simulink model "coupled_model"  (R2025b)
settings: Solver=ode4  StartTime=0.0  StopTime=20  FixedStep=0.01  RelTol=1e-3
InitFcn:
  | setup;
values from neighbouring files (symbols this model uses):
  K_GAIN = 1.0    (= 1)    [setup.m]
  N = 1000    [plot_out.m]    (also in setup.m)
  P_GAIN = 200.0    (= 200)    [setup.m]
  phase_offsets = [PHASE_OFFSET_RAD, -PHASE_OFFSET_RAD]    [setup.m]
  robot_params = struct()    [setup.m]
undefined symbols (not defined in the file or in its folder): tables1, tables2, X, Y, Z
libraries: sm_lib x30, nesl_utility x16
settings Model: Creator=mahdi  LastModifiedBy=root
settings SolverCC: AlgebraicLoopSolver=TrustRegion
settings DebuggingCC: UnconnectedInputMsg=warning  UnconnectedOutputMsg=warning  UnconnectedLineMsg=warning
settings ModelReferenceCC: EnableRefExpFcnMdlSchedulingChecks=on
settings RTWCC: GPUComputeCapability=3.5  DLArmComputeVersion=19.05

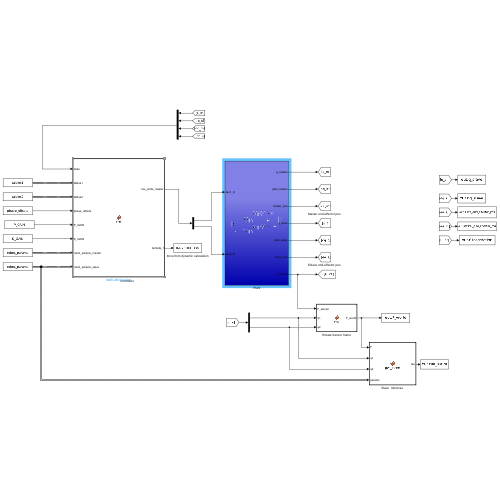
[thumbnail: Simulink's stored preview of the top-level diagram]
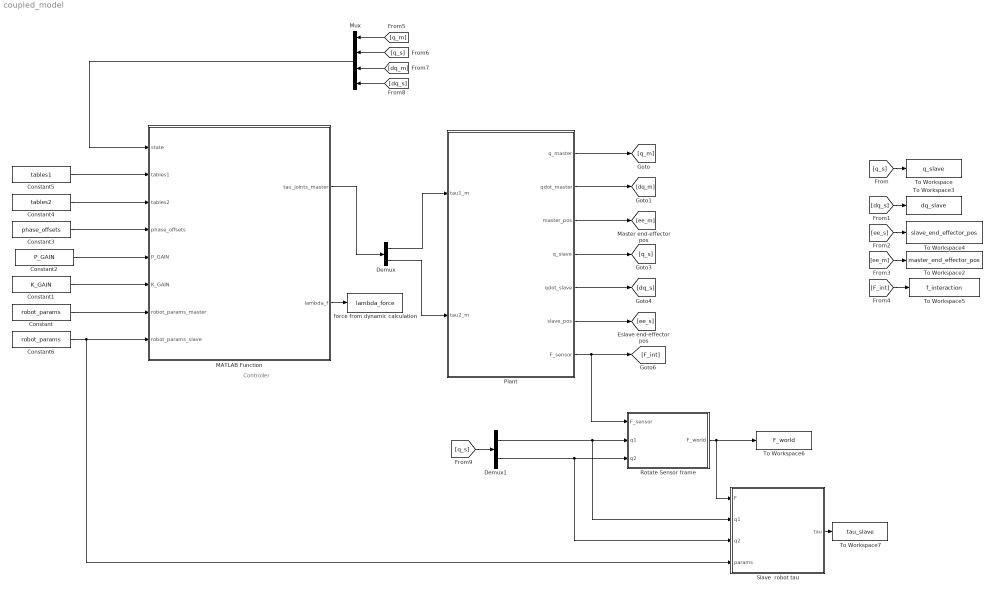
== system coupled_model ==
  note: Controller
  Constant : Constant  Value=robot_params  OutDataTypeStr=Bus: bus_RobotParams
  Constant1 : Constant  Value=K_GAIN
  Constant2 : Constant  Value=P_GAIN
  Constant3 : Constant  Value=phase_offsets
  Constant4 : Constant  Value=tables2  OutDataTypeStr=Bus: bus_Table
  Constant5 : Constant  Value=tables1  OutDataTypeStr=Bus:bus_Table
  Constant6 : Constant  Value=robot_params  OutDataTypeStr=Bus: bus_RobotParams
  Demux : Demux  Outputs=2
  Demux1 : Demux  Outputs=2
  MATLAB Function : MATLAB Function  TreatAsAtomicUnit=on
  Mux : Mux
  Plant : Subsystem
  Rotate Sensor frame : MATLAB Function  TreatAsAtomicUnit=on
  "Slave  robot tau " : MATLAB Function  TreatAsAtomicUnit=on
  To Workspace : ToWorkspace  VariableName=q_slave  SaveFormat=Timeseries  SampleTime=-1
  To Workspace2 : ToWorkspace  VariableName=master_end_effector_pos  SaveFormat=Timeseries  SampleTime=-1
  To Workspace3 : ToWorkspace  VariableName=dq_slave  SaveFormat=Timeseries  SampleTime=-1
  To Workspace4 : ToWorkspace  VariableName=slave_end_effector_pos  SaveFormat=Timeseries  SampleTime=-1
  To Workspace5 : ToWorkspace  VariableName=f_interaction  SaveFormat=Timeseries  SampleTime=-1
  To Workspace6 : ToWorkspace  VariableName=F_world  SaveFormat=Timeseries  SampleTime=-1
  To Workspace7 : ToWorkspace  VariableName=tau_slave  SaveFormat=Timeseries  SampleTime=-1
  force from dynamic calculation : ToWorkspace  VariableName=lambda_force  SaveFormat=Timeseries  SampleTime=-1
  wires:
  Constant5/1 -> MATLAB Function/2(tables1)
  Constant1/1 -> MATLAB Function/6(K_GAIN)
  Constant4/1 -> MATLAB Function/3(tables2)
  MATLAB Function/1(tau_joints_master) -> Demux/1
  Constant2/1 -> MATLAB Function/5(P_GAIN)
  Constant3/1 -> MATLAB Function/4(phase_offsets)
  Mux/1 -> MATLAB Function/1(state)
  Constant/1 -> MATLAB Function/7(robot_params_master)
  Constant6/1 -> "Slave  robot tau "/4(params), MATLAB Function/8(robot_params_slave)
  Demux/1 -> Plant/1(tau1_m)
  Demux/2 -> Plant/2(tau2_m)
  MATLAB Function/2(lambda_f) -> force from dynamic calculation/1
  Demux1/2 -> "Slave  robot tau "/3(q2), Rotate Sensor frame/3(q2)
  Demux1/1 -> "Slave  robot tau "/2(q1), Rotate Sensor frame/2(q1)
  Rotate Sensor frame/1(F_world) -> "Slave  robot tau "/1(F), To Workspace6/1
  "Slave  robot tau "/1(tau) -> To Workspace7/1
  Plant/1(q_master) -> [q_m]
  Plant/7(F_sensor) -> Rotate Sensor frame/1(F_sensor), [F_int]
  Plant/6(slave_pos) -> [ee_s]
  Plant/5(qdot_slave) -> [dq_s]
  Plant/4(q_slave) -> [q_s]
  Plant/2(qdot_master) -> [dq_m]
  Plant/3(master_pos) -> [ee_m]
  [q_s] -> To Workspace/1
  [dq_s] -> To Workspace3/1
  [ee_s] -> To Workspace4/1
  [ee_m] -> To Workspace2/1
  [F_int] -> To Workspace5/1
  [q_m] -> Mux/1
  [q_s] -> Mux/2
  [dq_m] -> Mux/3
  [dq_s] -> Mux/4
  [q_s] -> Demux1/1

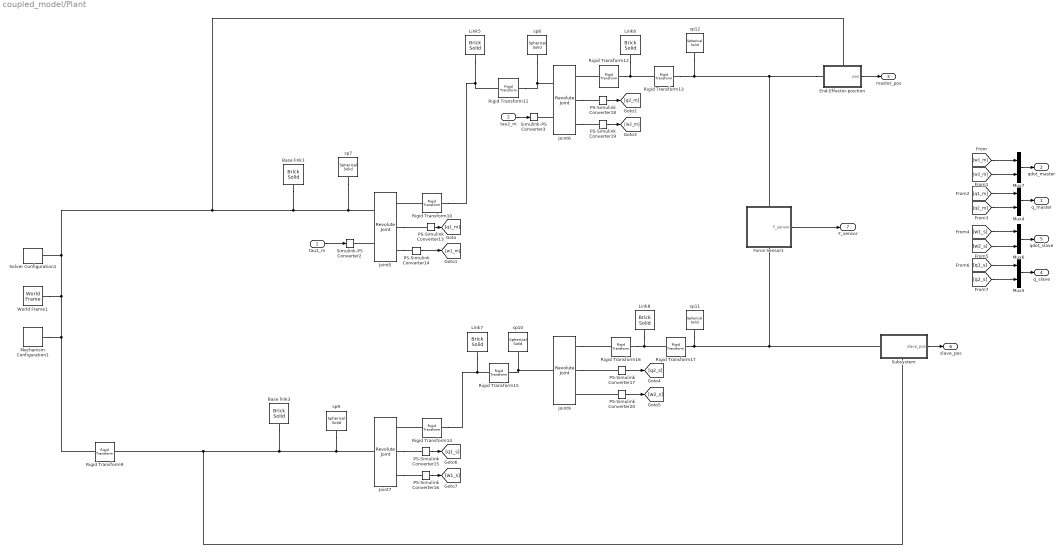
== system coupled_model/Plant ==
  tau1_m : Inport
  tau2_m : Inport  Port=2
  Base link1 : sm_lib/Body Elements/Brick Solid  BrickDimensions=[3 0.03 0.03]  BrickDimensionsUnits=m  ExportEntireGeometry=off  InertiaType=PointMass  BasedOnType=Density  Density=1000  DensityUnits=kg/m^3  Mass=0  MassUnits=kg  CenterOfMass=[0 0 0]  CenterOfMassUnits=m  MomentsOfInertia=[1 1 1]  MomentsOfInertiaUnits=kg*m^2  ProductsOfInertia=[0 0 0]  ProductsOfInertiaUnits=kg*m^2  GraphicType=FromGeometry  MarkerShape=Sphere  MarkerSize=10  GraphicVisPropType=SimpleVisualProperties  GraphicDiffuseColor=[0.2 0.0 0.2]  GraphicOpacity=1.0  GraphicSpecularColor=[0.5 0.5 0.5 1.0]  GraphicAmbientColor=[0.15 0.15 0.15 1.0]  GraphicEmissiveColor=[0.0 0.0 0.0 1.0]  GraphicShininess=75  DoExposeReferenceFrame=on  SerializedFrames=<Frames/>
  Base link3 : sm_lib/Body Elements/Brick Solid  BrickDimensions=[3 0.03 0.03]  BrickDimensionsUnits=m  ExportEntireGeometry=off  InertiaType=PointMass  BasedOnType=Density  Density=1000  DensityUnits=kg/m^3  Mass=0  MassUnits=kg  CenterOfMass=[0 0 0]  CenterOfMassUnits=m  MomentsOfInertia=[1 1 1]  MomentsOfInertiaUnits=kg*m^2  ProductsOfInertia=[0 0 0]  ProductsOfInertiaUnits=kg*m^2  GraphicType=FromGeometry  MarkerShape=Sphere  MarkerSize=10  GraphicVisPropType=SimpleVisualProperties  GraphicDiffuseColor=[0.2 0.0 0.2]  GraphicOpacity=1.0  GraphicSpecularColor=[0.5 0.5 0.5 1.0]  GraphicAmbientColor=[0.15 0.15 0.15 1.0]  GraphicEmissiveColor=[0.0 0.0 0.0 1.0]  GraphicShininess=75  DoExposeReferenceFrame=on  SerializedFrames=<Frames/>
  End-Effector-position : Subsystem
      settings: PortSchema="{\"entries\":[{\"content\":{\"sides\":[{\"content\":{\"connectorIds\":[\"LConn1\"]},\"type\":\"ConnectorPlacement.EquallySpacedRectSide\",\"uuid\":\"1bd7a165-eb29-492e-a5cd-16d291f82fae\"},{\"content\":{\"connectorIds\":[\"Out1\"],\"side\":\"RIGHT\"},\"type\":\"ConnectorPlacement.EquallySpacedRectSide\",\"uuid\":\"2a14fbc5-cc3d-44eb-82c9-5b5ff6534ee5\"},{\"content\":{\"connectorIds\":[\"LConn2\"],\"side\":\"TOP\"},\"type\":\"ConnectorPlacement.EquallySpacedRectSide\",\"uuid\":\"15682bf5-6b7b-4256-9b97-a5c9d4c612e4\"}]},\"type\":\"ConnectorPlacement.EquallySpacedConnector\",\"uuid\":\"8c85a081-e362-4ceb-b1e9-0f79b8921749\"}],\"packageUris\":[\"http://schema.mathworks.com/mf0/Connector/R2020b\"],\"version\":\"1.0\"}"
  Force Sensor1 : Subsystem
      settings: PortSchema="{\"entries\":[{\"content\":{\"sides\":[{\"content\":{},\"type\":\"ConnectorPlacement.EquallySpacedRectSide\",\"uuid\":\"1bd7a165-eb29-492e-a5cd-16d291f82fae\"},{\"content\":{\"connectorIds\":[\"Out1\"],\"side\":\"RIGHT\"},\"type\":\"ConnectorPlacement.EquallySpacedRectSide\",\"uuid\":\"2a14fbc5-cc3d-44eb-82c9-5b5ff6534ee5\"},{\"content\":{\"connectorIds\":[\"LConn1\"],\"side\":\"TOP\"},\"type\":\"ConnectorPlacement.EquallySpacedRectSide\",\"uuid\":\"15682bf5-6b7b-4256-9b97-a5c9d4c612e4\"},{\"content\":{\"connectorIds\":[\"RConn1\"],\"side\":\"BOTTOM\"},\"type\":\"ConnectorPlacement.EquallySpacedRectSide\",\"uuid\":\"076d02d1-429a-4e98-973e-cf78bfbce380\"}]},\"type\":\"ConnectorPlacement.EquallySpacedConnector\",\"uuid\":\"8c85a081-e362-4ceb-b1e9-0f79b8921749\"}],\"packageUris\":[\"http://schema.mathworks.com/mf0/Connector/R2020b\"],\"version\":\"1.0\"}"
  Joint5 : sm_lib/Joints/Revolute Joint  JointMode=Normal  CompositeWrenchDir=FollowerOnBase  CompositeWrenchFrame=BaseFrame  SenseConstraintForce=off  SenseConstraintTorque=off  SenseTotalForce=off  SenseTotalTorque=off  PositionTargetSpecify=on  PositionTargetPriority=High  PositionTargetValue=q1_m  PositionTargetValueUnits=rad  VelocityTargetSpecify=on  VelocityTargetPriority=High  VelocityTargetValue=0  VelocityTargetValueUnits=deg/s  EquilibriumPosition=0  EquilibriumPositionUnits=deg  SpringStiffness=0  SpringStiffnessUnits=N*m/deg  DampingCoefficient=0  DampingCoefficientUnits=N*m/(deg/s)  LowerLimitSpecify=off  LowerLimitBound=-90  LowerLimitBoundUnits=deg  LowerLimitStiffness=1e4  LowerLimitStiffnessUnits=N*m/deg  LowerLimitDamping=10  LowerLimitDampingUnits=N*m/(deg/s)  LowerLimitTransitionRegionWidth=0.1  LowerLimitTransitionRegionWidthUnits=deg  UpperLimitSpecify=off  UpperLimitBound=90  UpperLimitBoundUnits=deg  UpperLimitStiffness=1e4  UpperLimitStiffnessUnits=N*m/deg  UpperLimitDamping=10  UpperLimitDampingUnits=N*m/(deg/s)  UpperLimitTransitionRegionWidth=0.1  UpperLimitTransitionRegionWidthUnits=deg  TorqueActuationMode=InputTorque  MotionActuationMode=ComputedMotion  SensePosition=on  SenseVelocity=on  SenseAcceleration=off  SenseTorqueForce=off  SenseLowerLimitTorqueForce=off  SenseUpperLimitTorqueForce=off
  Joint6 : sm_lib/Joints/Revolute Joint  JointMode=Normal  CompositeWrenchDir=FollowerOnBase  CompositeWrenchFrame=BaseFrame  SenseConstraintForce=off  SenseConstraintTorque=off  SenseTotalForce=off  SenseTotalTorque=off  PositionTargetSpecify=on  PositionTargetPriority=High  PositionTargetValue=q2_m  PositionTargetValueUnits=rad  VelocityTargetSpecify=on  VelocityTargetPriority=High  VelocityTargetValue=0  VelocityTargetValueUnits=deg/s  EquilibriumPosition=0  EquilibriumPositionUnits=deg  SpringStiffness=0  SpringStiffnessUnits=N*m/deg  DampingCoefficient=0  DampingCoefficientUnits=N*m/(deg/s)  LowerLimitSpecify=off  LowerLimitBound=-90  LowerLimitBoundUnits=deg  LowerLimitStiffness=1e4  LowerLimitStiffnessUnits=N*m/deg  LowerLimitDamping=10  LowerLimitDampingUnits=N*m/(deg/s)  LowerLimitTransitionRegionWidth=0.1  LowerLimitTransitionRegionWidthUnits=deg  UpperLimitSpecify=off  UpperLimitBound=90  UpperLimitBoundUnits=deg  UpperLimitStiffness=1e4  UpperLimitStiffnessUnits=N*m/deg  UpperLimitDamping=10  UpperLimitDampingUnits=N*m/(deg/s)  UpperLimitTransitionRegionWidth=0.1  UpperLimitTransitionRegionWidthUnits=deg  TorqueActuationMode=InputTorque  MotionActuationMode=ComputedMotion  SensePosition=on  SenseVelocity=on  SenseAcceleration=off  SenseTorqueForce=off  SenseLowerLimitTorqueForce=off  SenseUpperLimitTorqueForce=off
  Joint7 : sm_lib/Joints/Revolute Joint  JointMode=Normal  CompositeWrenchDir=FollowerOnBase  CompositeWrenchFrame=BaseFrame  SenseConstraintForce=off  SenseConstraintTorque=off  SenseTotalForce=off  SenseTotalTorque=off  PositionTargetSpecify=on  PositionTargetPriority=High  PositionTargetValue=q1_s  PositionTargetValueUnits=rad  VelocityTargetSpecify=on  VelocityTargetPriority=High  VelocityTargetValue=0  VelocityTargetValueUnits=deg/s  EquilibriumPosition=0  EquilibriumPositionUnits=deg  SpringStiffness=0  SpringStiffnessUnits=N*m/deg  DampingCoefficient=0  DampingCoefficientUnits=N*m/(deg/s)  LowerLimitSpecify=off  LowerLimitBound=-90  LowerLimitBoundUnits=deg  LowerLimitStiffness=1e4  LowerLimitStiffnessUnits=N*m/deg  LowerLimitDamping=10  LowerLimitDampingUnits=N*m/(deg/s)  LowerLimitTransitionRegionWidth=0.1  LowerLimitTransitionRegionWidthUnits=deg  UpperLimitSpecify=off  UpperLimitBound=90  UpperLimitBoundUnits=deg  UpperLimitStiffness=1e4  UpperLimitStiffnessUnits=N*m/deg  UpperLimitDamping=10  UpperLimitDampingUnits=N*m/(deg/s)  UpperLimitTransitionRegionWidth=0.1  UpperLimitTransitionRegionWidthUnits=deg  TorqueActuationMode=NoTorque  MotionActuationMode=ComputedMotion  SensePosition=on  SenseVelocity=on  SenseAcceleration=off  SenseTorqueForce=off  SenseLowerLimitTorqueForce=off  SenseUpperLimitTorqueForce=off
  Joint9 : sm_lib/Joints/Revolute Joint  JointMode=Normal  CompositeWrenchDir=FollowerOnBase  CompositeWrenchFrame=BaseFrame  SenseConstraintForce=off  SenseConstraintTorque=off  SenseTotalForce=off  SenseTotalTorque=off  PositionTargetSpecify=on  PositionTargetPriority=High  PositionTargetValue=q2_s  PositionTargetValueUnits=rad  VelocityTargetSpecify=on  VelocityTargetPriority=High  VelocityTargetValue=0  VelocityTargetValueUnits=deg/s  EquilibriumPosition=0  EquilibriumPositionUnits=deg  SpringStiffness=0  SpringStiffnessUnits=N*m/deg  DampingCoefficient=0  DampingCoefficientUnits=N*m/(deg/s)  LowerLimitSpecify=off  LowerLimitBound=-90  LowerLimitBoundUnits=deg  LowerLimitStiffness=1e4  LowerLimitStiffnessUnits=N*m/deg  LowerLimitDamping=10  LowerLimitDampingUnits=N*m/(deg/s)  LowerLimitTransitionRegionWidth=0.1  LowerLimitTransitionRegionWidthUnits=deg  UpperLimitSpecify=off  UpperLimitBound=90  UpperLimitBoundUnits=deg  UpperLimitStiffness=1e4  UpperLimitStiffnessUnits=N*m/deg  UpperLimitDamping=10  UpperLimitDampingUnits=N*m/(deg/s)  UpperLimitTransitionRegionWidth=0.1  UpperLimitTransitionRegionWidthUnits=deg  TorqueActuationMode=NoTorque  MotionActuationMode=ComputedMotion  SensePosition=on  SenseVelocity=on  SenseAcceleration=off  SenseTorqueForce=off  SenseLowerLimitTorqueForce=off  SenseUpperLimitTorqueForce=off
  Link{5..8} (4 alike) : sm_lib/Body Elements/Brick Solid  BrickDimensions=[1 0.1 0.1]  BrickDimensionsUnits=m  ExportEntireGeometry=off  InertiaType=CalculateFromGeometry  BasedOnType=Mass  Density=7800  DensityUnits=kg/m^3  Mass=1  MassUnits=kg  CenterOfMass=[0 0 0]  CenterOfMassUnits=m  MomentsOfInertia=[1 1 1]  MomentsOfInertiaUnits=kg*m^2  ProductsOfInertia=[0 0 0]  ProductsOfInertiaUnits=kg*m^2  GraphicType=FromGeometry  MarkerShape=Sphere  MarkerSize=10  GraphicVisPropType=SimpleVisualProperties  GraphicDiffuseColor=[0.0 0.0 0.5]  GraphicOpacity=1.0  GraphicSpecularColor=[0.5 0.5 0.5 1.0]  GraphicAmbientColor=[0.15 0.15 0.15 1.0]  GraphicEmissiveColor=[0.0 0.0 0.0 1.0]  GraphicShininess=75  DoExposeReferenceFrame=on  SerializedFrames=<Frames/>
  Mechanism Configuration1 : sm_lib/Utilities/Mechanism Configuration  UniformGravity=Constant  GravityVector=[0 -9.81 0]  GravityVectorUnits=m/s^2  LinearizationDelta=0.001  JointModeTransitionNonlinearIterations=2
  Mux{4..7} (4 alike) : Mux  Inputs=2
  PS-Simulink Converter{13..20} (8 alike) : nesl_utility/PS-Simulink Converter  PhysicalDomain=network_engine_domain  SubClassName=ps_output  LeftPortType=input  RightPortType=output  PseudoPeriodic=off  Frequencies=[]  VectorFormat=1-D array  Unit=inherit  AffineConversion=off
  Rigid Transform{10..17} (8 alike) : sm_lib/Frames and Transforms/Rigid Transform  RotationMethod=None  FollAlignAxisA=+X  BaseAlignAxisA=+Y  FollAlignAxisB=+Y  BaseAlignAxisB=+Z  RotationStandardAxis=+Z  RotationAngle=0.0  RotationAngleUnits=deg  RotationArbitraryAxis=[0 0 1]  RotationSequenceAxes=FollowerAxes  RotationSequence=XYX  RotationSequenceAngles=[0 0 0]  RotationSequenceAnglesUnits=deg  RotationMatrix=[1 0 0; 0 1 0; 0 0 1]  Quaternion=[1 0 0 0]  TranslationMethod=StandardAxis  TranslationCartesianOffset=[0 0 0]  TranslationCartesianOffsetUnits=m  TranslationStandardAxis=+X  TranslationStandardOffset=0.5  TranslationStandardOffsetUnits=m  TranslationROffset=0  TranslationROffsetUnits=m  TranslationThetaOffset=0  TranslationThetaOffsetUnits=deg  TranslationZOffset=0  TranslationZOffsetUnits=m
  Rigid Transform9 : sm_lib/Frames and Transforms/Rigid Transform  RotationMethod=None  FollAlignAxisA=+X  BaseAlignAxisA=+Y  FollAlignAxisB=+Y  BaseAlignAxisB=+Z  RotationStandardAxis=+Z  RotationAngle=0.0  RotationAngleUnits=deg  RotationArbitraryAxis=[0 0 1]  RotationSequenceAxes=FollowerAxes  RotationSequence=XYX  RotationSequenceAngles=[0 0 0]  RotationSequenceAnglesUnits=deg  RotationMatrix=[1 0 0; 0 1 0; 0 0 1]  Quaternion=[1 0 0 0]  TranslationMethod=StandardAxis  TranslationCartesianOffset=[0 0 0]  TranslationCartesianOffsetUnits=m  TranslationStandardAxis=+X  TranslationStandardOffset=0  TranslationStandardOffsetUnits=m  TranslationROffset=0  TranslationROffsetUnits=m  TranslationThetaOffset=0  TranslationThetaOffsetUnits=deg  TranslationZOffset=0  TranslationZOffsetUnits=m
  Simulink-PS Converter2 : nesl_utility/Simulink-PS Converter  PhysicalDomain=network_engine_domain  SubClassName=ps_input  LeftPortType=input  RightPortType=output  PseudoPeriodic=off  Frequencies=[]  NoiseDistribution=none  NoiseParameters=[]  Unit=1  AffineConversion=off  FilteringAndDerivatives=provide  SimscapeFilterOrder=1  InputFilterTimeConstant=0.001  UdotUserProvided=0
  Simulink-PS Converter3 : nesl_utility/Simulink-PS Converter  PhysicalDomain=network_engine_domain  SubClassName=ps_input  LeftPortType=input  RightPortType=output  PseudoPeriodic=off  Frequencies=[]  NoiseDistribution=none  NoiseParameters=[]  Unit=1  AffineConversion=off  FilteringAndDerivatives=provide  SimscapeFilterOrder=1  InputFilterTimeConstant=0.001  UdotUserProvided=0
  Solver Configuration1 : nesl_utility/Solver Configuration  PhysicalDomain=network_engine_domain  SubClassName=solver  LeftPortType=input  RightPortType=generic  Tones=[]  Harmonics=[]  SimulateNoise=off  Profile=off  UseLocalSampling=off  EnableSwitchedLinearOptims=on  FrequencyDomain=off  UseCCode=off  RelTol=0.001  AbsTol=1e-06  MinStep=1e-09  ToWorkspace=off  RevertToSquareIcSolve=off  NumHomotopyIterations=100  PhasorMode=off  PhasorModeNumHarmonics=1  ConsistencySolver=NEWTON_FTOL  IndexReductionMethod=DerivativeReplacement  DoDC=off  ResidualTolerance=1e-09  ConsistencyTolSource=GLOBAL  ConsistencyAbsTol=0.001  ConsistencyRelTol=0.001  ConsistencyTolFactor=0.001  UseLocalSolver=off  LocalSolverChoice=NE_BACKWARD_EULER_ADVANCER  ResolveIndetEquations=on  FunctionEvalNumThread=1  LocalSolverSampleTime=0.001  DoFixedCost=off  MaxNonlinIter=3  MaxModeIter=2  ComputeImpulses=off  ImpulseIterations=2  LinearAlgebra=Sparse  LinearAlgebraNumThread=0  EquationFormulation=NE_TIME_EF  DelaysMemoryBudget=1024  AutomaticFiltering=on  FilteringTimeConstant=0.001  PartitionStorageMethod=AS_NEEDED  PartitionMemoryBudget=1024  PartitionMethod=FAST  MultibodyUseLocalSolver=off  MultibodyLocalSolverChoice=ODE1  MultibodyLocalSolverSampleTime=0.001
  Subsystem : Subsystem
      settings: PortSchema="{\"entries\":[{\"content\":{\"sides\":[{\"content\":{\"connectorIds\":[\"LConn1\"]},\"type\":\"ConnectorPlacement.EquallySpacedRectSide\",\"uuid\":\"741431ee-7711-4730-b4f3-6f21f1f2dad7\"},{\"content\":{\"connectorIds\":[\"Out1\"],\"side\":\"RIGHT\"},\"type\":\"ConnectorPlacement.EquallySpacedRectSide\",\"uuid\":\"25303491-3f58-4b32-a95a-180fbabe10d3\"},{\"content\":{\"side\":\"TOP\"},\"type\":\"ConnectorPlacement.EquallySpacedRectSide\",\"uuid\":\"22c9938c-adb9-4b64-a460-7b5d7d3f60d0\"},{\"content\":{\"connectorIds\":[\"RConn1\"],\"side\":\"BOTTOM\"},\"type\":\"ConnectorPlacement.EquallySpacedRectSide\",\"uuid\":\"15d6d459-f237-40cf-aebe-87cd9729afb5\"}]},\"type\":\"ConnectorPlacement.EquallySpacedConnector\",\"uuid\":\"9c6b3bf9-8c2e-46fa-81bd-189ed8538ab9\"}],\"packageUris\":[\"http://schema.mathworks.com/mf0/Connector/R2020b\"],\"version\":\"1.0\"}"
  World Frame1 : sm_lib/Frames and Transforms/World Frame
  sp10 : sm_lib/Body Elements/Spherical Solid  SphereRadius=0.08  SphereRadiusUnits=m  ExportEntireGeometry=off  InertiaType=PointMass  BasedOnType=Density  Density=1000  DensityUnits=kg/m^3  Mass=0  MassUnits=kg  CenterOfMass=[0 0 0]  CenterOfMassUnits=m  MomentsOfInertia=[1 1 1]  MomentsOfInertiaUnits=kg*m^2  ProductsOfInertia=[0 0 0]  ProductsOfInertiaUnits=kg*m^2  GraphicType=FromGeometry  MarkerShape=Sphere  MarkerSize=10  GraphicVisPropType=SimpleVisualProperties  GraphicDiffuseColor=[0 0.3333 0]  GraphicOpacity=1.0  GraphicSpecularColor=[0.5 0.5 0.5 1.0]  GraphicAmbientColor=[0.15 0.15 0.15 1.0]  GraphicEmissiveColor=[0.0 0.0 0.0 1.0]  GraphicShininess=75  DoExposeReferenceFrame=on  SerializedFrames=<Frames/>
  sp11 : sm_lib/Body Elements/Spherical Solid  SphereRadius=0.08  SphereRadiusUnits=m  ExportEntireGeometry=off  InertiaType=PointMass  BasedOnType=Density  Density=1000  DensityUnits=kg/m^3  Mass=0  MassUnits=kg  CenterOfMass=[0 0 0]  CenterOfMassUnits=m  MomentsOfInertia=[1 1 1]  MomentsOfInertiaUnits=kg*m^2  ProductsOfInertia=[0 0 0]  ProductsOfInertiaUnits=kg*m^2  GraphicType=FromGeometry  MarkerShape=Sphere  MarkerSize=10  GraphicVisPropType=SimpleVisualProperties  GraphicDiffuseColor=[0 0.3333 0]  GraphicOpacity=1.0  GraphicSpecularColor=[0.5 0.5 0.5 1.0]  GraphicAmbientColor=[0.15 0.15 0.15 1.0]  GraphicEmissiveColor=[0.0 0.0 0.0 1.0]  GraphicShininess=75  DoExposeReferenceFrame=on  SerializedFrames=<Frames/>
  sp12 : sm_lib/Body Elements/Spherical Solid  SphereRadius=0.08  SphereRadiusUnits=m  ExportEntireGeometry=off  InertiaType=PointMass  BasedOnType=Density  Density=1000  DensityUnits=kg/m^3  Mass=0  MassUnits=kg  CenterOfMass=[0 0 0]  CenterOfMassUnits=m  MomentsOfInertia=[1 1 1]  MomentsOfInertiaUnits=kg*m^2  ProductsOfInertia=[0 0 0]  ProductsOfInertiaUnits=kg*m^2  GraphicType=FromGeometry  MarkerShape=Sphere  MarkerSize=10  GraphicVisPropType=SimpleVisualProperties  GraphicDiffuseColor=[0.2 1.0 0.2]  GraphicOpacity=1.0  GraphicSpecularColor=[0.5 0.5 0.5 1.0]  GraphicAmbientColor=[0.15 0.15 0.15 1.0]  GraphicEmissiveColor=[0.0 0.0 0.0 1.0]  GraphicShininess=75  DoExposeReferenceFrame=on  SerializedFrames=<Frames/>
  sp7 : sm_lib/Body Elements/Spherical Solid  SphereRadius=0.08  SphereRadiusUnits=m  ExportEntireGeometry=off  InertiaType=PointMass  BasedOnType=Density  Density=1000  DensityUnits=kg/m^3  Mass=0  MassUnits=kg  CenterOfMass=[0 0 0]  CenterOfMassUnits=m  MomentsOfInertia=[1 1 1]  MomentsOfInertiaUnits=kg*m^2  ProductsOfInertia=[0 0 0]  ProductsOfInertiaUnits=kg*m^2  GraphicType=FromGeometry  MarkerShape=Sphere  MarkerSize=10  GraphicVisPropType=SimpleVisualProperties  GraphicDiffuseColor=[0.9 0.0 0.0]  GraphicOpacity=1.0  GraphicSpecularColor=[0.5 0.5 0.5 1.0]  GraphicAmbientColor=[0.15 0.15 0.15 1.0]  GraphicEmissiveColor=[0.0 0.0 0.0 1.0]  GraphicShininess=75  DoExposeReferenceFrame=on  SerializedFrames=<Frames/>
  sp8 : sm_lib/Body Elements/Spherical Solid  SphereRadius=0.08  SphereRadiusUnits=m  ExportEntireGeometry=off  InertiaType=PointMass  BasedOnType=Density  Density=1000  DensityUnits=kg/m^3  Mass=0  MassUnits=kg  CenterOfMass=[0 0 0]  CenterOfMassUnits=m  MomentsOfInertia=[1 1 1]  MomentsOfInertiaUnits=kg*m^2  ProductsOfInertia=[0 0 0]  ProductsOfInertiaUnits=kg*m^2  GraphicType=FromGeometry  MarkerShape=Sphere  MarkerSize=10  GraphicVisPropType=SimpleVisualProperties  GraphicDiffuseColor=[0.9 0.0 0.0]  GraphicOpacity=1.0  GraphicSpecularColor=[0.5 0.5 0.5 1.0]  GraphicAmbientColor=[0.15 0.15 0.15 1.0]  GraphicEmissiveColor=[0.0 0.0 0.0 1.0]  GraphicShininess=75  DoExposeReferenceFrame=on  SerializedFrames=<Frames/>
  sp9 : sm_lib/Body Elements/Spherical Solid  SphereRadius=0.08  SphereRadiusUnits=m  ExportEntireGeometry=off  InertiaType=PointMass  BasedOnType=Density  Density=1000  DensityUnits=kg/m^3  Mass=0  MassUnits=kg  CenterOfMass=[0 0 0]  CenterOfMassUnits=m  MomentsOfInertia=[1 1 1]  MomentsOfInertiaUnits=kg*m^2  ProductsOfInertia=[0 0 0]  ProductsOfInertiaUnits=kg*m^2  GraphicType=FromGeometry  MarkerShape=Sphere  MarkerSize=10  GraphicVisPropType=SimpleVisualProperties  GraphicDiffuseColor=[0 0.3333 0]  GraphicOpacity=1.0  GraphicSpecularColor=[0.5 0.5 0.5 1.0]  GraphicAmbientColor=[0.15 0.15 0.15 1.0]  GraphicEmissiveColor=[0.0 0.0 0.0 1.0]  GraphicShininess=75  DoExposeReferenceFrame=on  SerializedFrames=<Frames/>
  q_master : Outport
  qdot_master : Outport  Port=2
  master_pos : Outport  Port=3
  q_slave : Outport  Port=4
  qdot_slave : Outport  Port=5
  slave_pos : Outport  Port=6
  F_sensor : Outport  Port=7
  wires:
  PS-Simulink Converter20/1 -> [w2_s]
  Mux5/1 -> q_slave/1
  [q1_s] -> Mux5/1
  [w1_s] -> Mux6/1
  [q2_m] -> Mux4/2
  Subsystem/1(slave_pos) -> slave_pos/1
  [w2_s] -> Mux6/2
  [q1_m] -> Mux4/1
  [q2_s] -> Mux5/2
  PS-Simulink Converter16/1 -> [w1_s]
  Mux7/1 -> qdot_master/1
  PS-Simulink Converter14/1 -> [w1_m]
  [w1_m] -> Mux7/1
  Mux4/1 -> q_master/1
  [w2_m] -> Mux7/2
  PS-Simulink Converter13/1 -> [q1_m]
  PS-Simulink Converter19/1 -> [w2_m]
  tau2_m/1 -> Simulink-PS Converter3/1
  PS-Simulink Converter18/1 -> [q2_m]
  Force Sensor1/1(F_sensor) -> F_sensor/1
  tau1_m/1 -> Simulink-PS Converter2/1
  PS-Simulink Converter15/1 -> [q1_s]
  End-Effector-position/1(pos) -> master_pos/1
  Mux6/1 -> qdot_slave/1
  PS-Simulink Converter17/1 -> [q2_s]
  connections:
  Rigid Transform12/RConn1 -- Link6/RConn1 -- Rigid Transform13/LConn1
  End-Effector-position/LConn1 -- sp12/RConn1 -- Rigid Transform13/RConn1 -- Force Sensor1/LConn1
  Rigid Transform9/RConn1 -- Subsystem/RConn1 -- Joint7/LConn1 -- sp9/RConn1 -- Base link3/RConn1
  Rigid Transform15/RConn1 -- Joint9/LConn1 -- sp10/RConn1
  Force Sensor1/RConn1 -- Subsystem/LConn1 -- sp11/RConn1 -- Rigid Transform17/RConn1
  End-Effector-position/LConn2 -- Mechanism Configuration1/RConn1 -- Rigid Transform9/LConn1 -- World Frame1/RConn1 -- Solver Configuration1/RConn1 -- Base link1/RConn1 -- Joint5/LConn1 -- sp7/RConn1
  Rigid Transform16/RConn1 -- Rigid Transform17/LConn1 -- Link8/RConn1
  Rigid Transform10/RConn1 -- Link5/RConn1 -- Rigid Transform11/LConn1
  Rigid Transform14/RConn1 -- Link7/RConn1 -- Rigid Transform15/LConn1
  Rigid Transform11/RConn1 -- Joint6/LConn1 -- sp8/RConn1
  Joint5/RConn2 -- PS-Simulink Converter13/LConn1
  Joint6/RConn2 -- PS-Simulink Converter18/LConn1
  Joint7/RConn2 -- PS-Simulink Converter15/LConn1
  Joint6/RConn3 -- PS-Simulink Converter19/LConn1
  PS-Simulink Converter20/LConn1 -- Joint9/RConn3
  Joint5/RConn3 -- PS-Simulink Converter14/LConn1
  Rigid Transform12/LConn1 -- Joint6/RConn1
  Joint9/RConn1 -- Rigid Transform16/LConn1
  Joint7/RConn3 -- PS-Simulink Converter16/LConn1
  Joint6/LConn2 -- Simulink-PS Converter3/RConn1
  Joint5/LConn2 -- Simulink-PS Converter2/RConn1
  Rigid Transform10/LConn1 -- Joint5/RConn1
  Rigid Transform14/LConn1 -- Joint7/RConn1
  Joint9/RConn2 -- PS-Simulink Converter17/LConn1

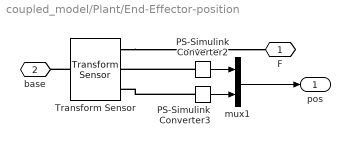
== system coupled_model/Plant/End-Effector-position ==
  PS-Simulink Converter2 : nesl_utility/PS-Simulink Converter  PhysicalDomain=network_engine_domain  SubClassName=ps_output  LeftPortType=input  RightPortType=output  PseudoPeriodic=off  Frequencies=[]  VectorFormat=1-D array  Unit=inherit  AffineConversion=off
  PS-Simulink Converter3 : nesl_utility/PS-Simulink Converter  PhysicalDomain=network_engine_domain  SubClassName=ps_output  LeftPortType=input  RightPortType=output  PseudoPeriodic=off  Frequencies=[]  VectorFormat=1-D array  Unit=inherit  AffineConversion=off
  Transform Sensor : sm_lib/Frames and Transforms/Transform Sensor  MeasurementFrame=World  RotationSequence=XYX  SenseAngle=off  SenseAxis=off  SenseQ=off  SenseR=off  SenseRotationSequence=off  SenseOmegaX=off  SenseOmegaY=off  SenseOmegaZ=off  SenseOmega=off  SenseQDot=off  SenseRDot=off  SenseRotationSequenceDot=off  SenseAlphaX=off  SenseAlphaY=off  SenseAlphaZ=off  SenseAlpha=off  SenseQDDot=off  SenseRDDot=off  SenseX=on  SenseY=on  SenseZ=off  SenseXYZ=off  SenseRad=off  SenseAzim=off  SenseDist=off  SenseInc=off  SenseXDot=off  SenseYDot=off  SenseZDot=off  SenseXYZDot=off  SenseRadDot=off  SenseAzimDot=off  SenseDistDot=off  SenseIncDot=off  SenseXDDot=off  SenseYDDot=off  SenseZDDot=off  SenseXYZDDot=off  SenseRadDDot=off  SenseAzimDDot=off  SenseDistDDot=off  SenseIncDDot=off
  mux1 : Mux  Inputs=2
  F : PMIOPort  Side=Left
  base : PMIOPort  Port=2  Side=Left
  pos : Outport
  wires:
  PS-Simulink Converter3/1 -> mux1/2
  PS-Simulink Converter2/1 -> mux1/1
  mux1/1 -> pos/1
  connections:
  PS-Simulink Converter2/LConn1 -- Transform Sensor/RConn2
  Transform Sensor/RConn1 -- F/RConn1
  PS-Simulink Converter3/LConn1 -- Transform Sensor/RConn3
  Transform Sensor/LConn1 -- base/RConn1

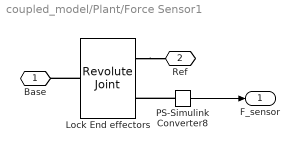
== system coupled_model/Plant/Force Sensor1 ==
  Lock End effectors : sm_lib/Joints/Revolute Joint  JointMode=Normal  CompositeWrenchDir=FollowerOnBase  CompositeWrenchFrame=FollowerFrame  SenseConstraintForce=on  SenseConstraintTorque=off  SenseTotalForce=off  SenseTotalTorque=off  PositionTargetSpecify=off  PositionTargetPriority=High  PositionTargetValue=0  PositionTargetValueUnits=deg  VelocityTargetSpecify=off  VelocityTargetPriority=High  VelocityTargetValue=0  VelocityTargetValueUnits=deg/s  EquilibriumPosition=0  EquilibriumPositionUnits=deg  SpringStiffness=0  SpringStiffnessUnits=N*m/deg  DampingCoefficient=0  DampingCoefficientUnits=N*m/(deg/s)  LowerLimitSpecify=off  LowerLimitBound=-90  LowerLimitBoundUnits=deg  LowerLimitStiffness=1e4  LowerLimitStiffnessUnits=N*m/deg  LowerLimitDamping=10  LowerLimitDampingUnits=N*m/(deg/s)  LowerLimitTransitionRegionWidth=0.1  LowerLimitTransitionRegionWidthUnits=deg  UpperLimitSpecify=off  UpperLimitBound=90  UpperLimitBoundUnits=deg  UpperLimitStiffness=1e4  UpperLimitStiffnessUnits=N*m/deg  UpperLimitDamping=10  UpperLimitDampingUnits=N*m/(deg/s)  UpperLimitTransitionRegionWidth=0.1  UpperLimitTransitionRegionWidthUnits=deg  TorqueActuationMode=NoTorque  MotionActuationMode=ComputedMotion  SensePosition=off  SenseVelocity=off  SenseAcceleration=off  SenseTorqueForce=off  SenseLowerLimitTorqueForce=off  SenseUpperLimitTorqueForce=off
  PS-Simulink Converter8 : nesl_utility/PS-Simulink Converter  PhysicalDomain=network_engine_domain  SubClassName=ps_output  LeftPortType=input  RightPortType=output  PseudoPeriodic=off  Frequencies=[]  VectorFormat=inherit  Unit=inherit  AffineConversion=off
  Base : PMIOPort  Side=Left
  Ref : PMIOPort  Port=2  Side=Right
  F_sensor : Outport
  wires:
  PS-Simulink Converter8/1 -> F_sensor/1
  connections:
  Lock End effectors/RConn1 -- Ref/RConn1
  Lock End effectors/LConn1 -- Base/RConn1
  PS-Simulink Converter8/LConn1 -- Lock End effectors/RConn2

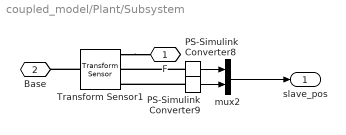
== system coupled_model/Plant/Subsystem ==
  PS-Simulink Converter8 : nesl_utility/PS-Simulink Converter  PhysicalDomain=network_engine_domain  SubClassName=ps_output  LeftPortType=input  RightPortType=output  PseudoPeriodic=off  Frequencies=[]  VectorFormat=1-D array  Unit=inherit  AffineConversion=off
  PS-Simulink Converter9 : nesl_utility/PS-Simulink Converter  PhysicalDomain=network_engine_domain  SubClassName=ps_output  LeftPortType=input  RightPortType=output  PseudoPeriodic=off  Frequencies=[]  VectorFormat=1-D array  Unit=inherit  AffineConversion=off
  Transform Sensor1 : sm_lib/Frames and Transforms/Transform Sensor  MeasurementFrame=World  RotationSequence=XYX  SenseAngle=off  SenseAxis=off  SenseQ=off  SenseR=off  SenseRotationSequence=off  SenseOmegaX=off  SenseOmegaY=off  SenseOmegaZ=off  SenseOmega=off  SenseQDot=off  SenseRDot=off  SenseRotationSequenceDot=off  SenseAlphaX=off  SenseAlphaY=off  SenseAlphaZ=off  SenseAlpha=off  SenseQDDot=off  SenseRDDot=off  SenseX=on  SenseY=on  SenseZ=off  SenseXYZ=off  SenseRad=off  SenseAzim=off  SenseDist=off  SenseInc=off  SenseXDot=off  SenseYDot=off  SenseZDot=off  SenseXYZDot=off  SenseRadDot=off  SenseAzimDot=off  SenseDistDot=off  SenseIncDot=off  SenseXDDot=off  SenseYDDot=off  SenseZDDot=off  SenseXYZDDot=off  SenseRadDDot=off  SenseAzimDDot=off  SenseDistDDot=off  SenseIncDDot=off
  mux2 : Mux  Inputs=2
  F : PMIOPort  Side=Left
  Base : PMIOPort  Port=2  Side=Right
  slave_pos : Outport
  wires:
  PS-Simulink Converter8/1 -> mux2/1
  PS-Simulink Converter9/1 -> mux2/2
  mux2/1 -> slave_pos/1
  connections:
  Transform Sensor1/LConn1 -- Base/RConn1
  PS-Simulink Converter9/LConn1 -- Transform Sensor1/RConn3
  PS-Simulink Converter8/LConn1 -- Transform Sensor1/RConn2
  Transform Sensor1/RConn1 -- F/RConn1

== matlab function coupled_model/Rotate Sensor frame ==
  data: F_sensor input; F_world output; q1 input; q2 input
function F_world = fcn(F_sensor, q1, q2)
    theta_total = q1 + q2; 
    
    R = [cos(theta_total), -sin(theta_total);
         sin(theta_total),  cos(theta_total)];
    
    F_world = R * F_sensor(1:2, :);

== matlab function coupled_model/MATLAB Function ==
  data: state input; tables1 input; tau_joints_master output; tables2 input; phase_offsets input; P_GAIN input; K_GAIN input; robot_params_master input; robot_params_slave input; lambda_f output
function [tau_joints_master, lambda_f] = fcn(state, tables1, tables2, phase_offsets, P_GAIN, K_GAIN, robot_params_master, robot_params_slave)
    
    q_master = state(1:2);       
    q_slave  = state(3:4);       
    q_dot_master = state(5:6);   
    q_dot_slave  = state(7:8);   
    
    % Master kinematics and Jacobian
    [x_master, y_master] = forward_kinematics(q_master(1), q_master(2), robot_params_master);
    J_master = get_jacob(q_master(1), q_master(2), robot_params_master);
    J_dot_master = get_jacob_dot(q_master(1), q_master(2), q_dot_master, robot_params_master);
    
    vel_master_cart = J_master * q_dot_master; 
    master_x_axis_state = [x_master; vel_master_cart(1)];
    master_y_axis_state = [y_master; vel_master_cart(2)];
    
    % Phase calculation
    x_pitch = get_pitch(master_x_axis_state, tables1);
    y_pitch = get_pitch(master_y_axis_state, tables2);
    
    % VER controller target accelerations
    xddot_ver = get_desired_acceleration(master_x_axis_state, y_pitch, phase_offsets(1), tables1, P_GAIN, K_GAIN);  
    yddot_ver = get_desired_acceleration(master_y_axis_state, x_pitch, phase_offsets(2), tables2, P_GAIN, K_GAIN); 
    desired_acc = [xddot_ver; yddot_ver];
    
    % Slave dynamics and Jacobian
    [M_slave, CG_slave] = compute_distributed_mass_dynamics(q_slave, q_dot_slave, robot_params_slave);
    J_slave = get_jacob(q_slave(1), q_slave(2), robot_params_slave);
    J_dot_slave = get_jacob_dot(q_slave(1), q_slave(2), q_dot_slave, robot_params_slave);
    
    % Master dynamics
    [M_master, CG_master] = compute_distributed_mass_dynamics(q_master, q_dot_master, robot_params_master);
    
    % Linear system formulation: [qdd_m; qdd_s; lambda; tau_m]
    z2 = zeros(2, 2);
    i2 = eye(2);
    
    coef_matrix = [
        J_master, z2,       z2,        z2;
        z2,       J_slave,  z2,        z2;
        z2,       M_slave,  -J_slave', z2;
        M_master, z2,       J_master', -i2
    ];
    
    b_matrix = [
        desired_acc - (J_dot_master * q_dot_master);
        desired_acc - (J_dot_slave * q_dot_slave);
        -CG_slave;
        -CG_master
    ];
    
    control_solution = coef_matrix \ b_matrix;
    
    lambda_f = control_solution(5:6);
    tau_joints_master = control_solution(7:8);
end

function u_ver = get_desired_acceleration(current_state, other_joint_pitch, phase_offset_rad, table, P, K)
    x = current_state(1);
    x_dot = current_state(2);
    x_centered = x - table.center;
    
    current_theta = atan2(x_dot, x_centered);
    current_r_sq = x_centered^2 + x_dot^2;
    
    min_theta = table.theta(1); 
    max_theta = table.theta(end);
    current_theta_interp = min_theta + mod(current_theta - min_theta, max_theta - min_theta);
    
    desired_r_d = interp1(table.theta, table.r_d, current_theta_interp, 'linear');
    beta = interp1(table.theta, table.beta, current_theta_interp, 'linear');
    
    current_pitch = get_pitch(current_state, table); 
    
    alpha = P * tanh(x_dot) * (desired_r_d^2 - current_r_sq);
    gamma = K * (sin(other_joint_pitch + phase_offset_rad) - sin(current_pitch));
    
    u_ver = alpha + beta + gamma;
end

function current_pitch = get_pitch(current_state, table)
    current_pitch = atan2(current_state(2), current_state(1) - table.center);
end

function [M, CG] = compute_distributed_mass_dynamics(q, q_dot, params)
    l1 = params.L1; l2 = params.L2; 
    m1 = params.m1; m2 = params.m2; 
    I1 = params.I1; I2 = params.I2; 
    g = params.g;
    
    q1 = q(1); q2 = q(2); 
    dq1 = q_dot(1); dq2 = q_dot(2); 
    
    d11 = I1 + I2 + (m2*((l2*cos(q1 + q2) + 2*l1*cos(q1))*((l2*cos(q1 + q2))/2 + l1*cos(q1)) + (l2*sin(q1 + q2) + 2*l1*sin(q1))*((l2*sin(q1 + q2))/2 + l1*sin(q1))))/2 + (m1*((l1^2*cos(q1)^2)/2 + (l1^2*sin(q1)^2)/2))/2;
    d12 = I2 + (m2*(l2*sin(q1 + q2)*((l2*sin(q1 + q2))/2 + l1*sin(q1)) + l2*cos(q1 + q2)*((l2*cos(q1 + q2))/2 + l1*cos(q1))))/2;
    d22 = I2 + (m2*((l2^2*cos(q1 + q2)^2)/2 + (l2^2*sin(q1 + q2)^2)/2))/2;
    M = [d11, d12; d12, d22];
    
    % dx and dy terms removed as they are analytically zero
    cg1 = ((m2*((dq1*l1*cos(q1) + (l2*cos(q1 + q2)*(dq1 + dq2))/2)*(2*dq1*l1*sin(q1) + l2*sin(q1 + q2)*(dq1 + dq2)) - (dq1*l1*sin(q1) + (l2*sin(q1 + q2)*(dq1 + dq2))/2)*(2*dq1*l1*cos(q1) + l2*cos(q1 + q2)*(dq1 + dq2)) - ((l2*cos(q1 + q2))/2 + l1*cos(q1))*(l2*sin(q1 + q2)*(dq1 + dq2)^2 + 2*dq1^2*l1*sin(q1)) + ((l2*sin(q1 + q2))/2 + l1*sin(q1))*(2*dq1^2*l1*cos(q1) + l2*cos(q1 + q2)*(dq1 + dq2)^2)))/2 - (m2*((dq1*l1*cos(q1) + (l2*cos(q1 + q2)*(dq1 + dq2))/2)*(2*dq1*l1*sin(q1) + l2*sin(q1 + q2)*(dq1 + dq2)) - (dq1*l1*sin(q1) + (l2*sin(q1 + q2)*(dq1 + dq2))/2)*(2*dq1*l1*cos(q1) + l2*cos(q1 + q2)*(dq1 + dq2))))/2 + g*m2*((l2*cos(q1 + q2))/2 + l1*cos(q1)) + (g*l1*m1*cos(q1))/2);
    cg2 = ((m2*(l2*sin(q1 + q2)*(dq1^2*l1*cos(q1) + (l2*cos(q1 + q2)*(dq1 + dq2)^2)/2) - l2*cos(q1 + q2)*((l2*sin(q1 + q2)*(dq1 + dq2)^2)/2 + dq1^2*l1*sin(q1)) - l2*sin(q1 + q2)*(dq1 + dq2)*(dq1*l1*cos(q1) + (l2*cos(q1 + q2)*(dq1 + dq2))/2) + l2*cos(q1 + q2)*(dq1 + dq2)*(dq1*l1*sin(q1) + (l2*sin(q1 + q2)*(dq1 + dq2))/2)))/2 + (m2*(l2*sin(q1 + q2)*(dq1 + dq2)*(dq1*l1*cos(q1) + (l2*cos(q1 + q2)*(dq1 + dq2))/2) - l2*cos(q1 + q2)*(dq1 + dq2)*(dq1*l1*sin(q1) + (l2*sin(q1 + q2)*(dq1 + dq2))/2)))/2 + (g*l2*m2*cos(q1 + q2))/2);
    CG = [cg1; cg2];
end

function [x, y] = forward_kinematics(q1, q2, params)
    x = params.L1 * cos(q1) + params.L2 * cos(q1 + q2);
    y = params.L1 * sin(q1) + params.L2 * sin(q1 + q2);
end

function J = get_jacob(q1, q2, params)
    s1 = sin(q1); c1 = cos(q1); s12 = sin(q1 + q2); c12 = cos(q1 + q2);
    J = [-params.L1*s1 - params.L2*s12, -params.L2*s12;
          params.L1*c1 + params.L2*c12,  params.L2*c12];
end
    
function Jdot = get_jacob_dot(q1, q2, q_dot, params)
    l1 = params.L1; l2 = params.L2; 
    c1 = cos(q1); s1 = sin(q1); 
    c12 = cos(q1 + q2); s12 = sin(q1 + q2); 
    dq_sum = q_dot(1) + q_dot(2);
    
    Jdot = [-l1*c1*q_dot(1) - l2*c12*dq_sum, -l2*c12*dq_sum; 
            -l1*s1*q_dot(1) - l2*s12*dq_sum, -l2*s12*dq_sum];
end

== matlab function coupled_model/Slave  robot tau  ==
  data: F input; q1 input; tau output; q2 input; params input
function tau = get_jacob(F, q1, q2, params)
    s1 = sin(q1); c1 = cos(q1); s12 = sin(q1 + q2); c12 = cos(q1 + q2);
    J = [-params.L1*s1 - params.L2*s12, -params.L2*s12;
          params.L1*c1 + params.L2*c12,  params.L2*c12];

    tau = J'*F;
end
